simulink model "sysgenCORDICSinCos"  (Simulink 7.7)
settings: Solver=ode45  StartTime=0.0  StopTime=500  RelTol=1e-3
values from neighbouring files (symbols this model uses):
  blue = blue(1:(min_x*min_y))    [makematrix.m]    (also in rgb.mat = [0 0 0 255 255 255 255 255 255 0 0 0 ... (256 elements, 256x)
undefined symbols (not defined in the file or in its folder): Error_Measurement, sysgenCORDIC_lib
libraries: xbsIndex_r4 x95, dspobslib x9, dspstat3 x4, dspswit3 x2, xbsCopyrightNotice_r4 x1, simulink x1
(part 2 of 2)

== system sysgenCORDICSinCos/SINCOS testbench/SinCos/fine_angle_pe/cordic_pe7 ==
  xi : Inport
  yi : Inport  Port=2
  zi : Inport  Port=3
  AddSub22 : xbsIndex_r4/AddSub  mode=Addition or Subtraction  use_carryin=off  use_carryout=off  en=off  latency=1  precision=User Defined  arith_type="Signed  (2's comp)"  n_bits=16  bin_pt=13  quantization=Truncate  overflow=Wrap  dbl_ovrd=off  use_behavioral_HDL=off  hw_selection=Fabric  pipelined=off  block_type=addsub
  AddSub23 : xbsIndex_r4/AddSub  mode=Addition or Subtraction  use_carryin=off  use_carryout=off  en=off  latency=1  precision=User Defined  arith_type="Signed  (2's comp)"  n_bits=16  bin_pt=13  quantization=Truncate  overflow=Wrap  dbl_ovrd=off  use_behavioral_HDL=off  hw_selection=Fabric  pipelined=off  block_type=addsub
  AddSub24 : xbsIndex_r4/AddSub  mode=Addition or Subtraction  use_carryin=off  use_carryout=off  en=off  latency=1  precision=User Defined  arith_type="Signed  (2's comp)"  n_bits=16  bin_pt=13  quantization=Truncate  overflow=Wrap  dbl_ovrd=off  use_behavioral_HDL=off  hw_selection=Fabric  pipelined=off  block_type=addsub
  Constant11 : xbsIndex_r4/Constant  const=0.00781234106010111  gui_display_data_type=Fixed-point  arith_type=Signed (2's comp)  n_bits=16  bin_pt=13  preci_type=Single  exp_width=8  frac_width=24  explicit_period=off  period=1  equ=P=C  opselect=C  inp2=PCIN>>17  opr=+  inp1=P  carry=CIN  dbl_ovrd=off  block_type=constant
  Inverter8 : xbsIndex_r4/Inverter  en=off  latency=0  dbl_ovrd=off  block_type=inv
  Shift14 : xbsIndex_r4/Shift  shift_dir=Right  shift_bits=7  en=off  latency=0  precision=User Defined  arith_type="Signed  (2's comp)"  n_bits=16  bin_pt=13  quantization=Truncate  overflow=Wrap  dbl_ovrd=off  block_type=shift
  Shift15 : xbsIndex_r4/Shift  shift_dir=Right  shift_bits=7  en=off  latency=0  precision=User Defined  arith_type="Signed  (2's comp)"  n_bits=16  bin_pt=13  quantization=Truncate  overflow=Wrap  dbl_ovrd=off  block_type=shift
  Slice9 : xbsIndex_r4/Slice  nbits=1  boolean_output=on  mode=Upper Bit Location + Width  bit1=0  base1=MSB of Input  bit0=0  base0=LSB of Input  dbl_ovrd=off  block_type=slice
  xo : Outport
  yo : Outport  Port=2
  zo : Outport  Port=3
  wires:
  xi/1 -> AddSub22/1, Shift14/1
  yi/1 -> AddSub23/1, Shift15/1
  zi/1 -> AddSub24/1, Slice9/1
  Slice9/1 -> AddSub23/3, Inverter8/1
  Inverter8/1 -> AddSub24/3, AddSub22/3
  AddSub24/1 -> zo/1
  Constant11/1 -> AddSub24/2
  AddSub23/1 -> yo/1
  Shift14/1 -> AddSub23/2
  AddSub22/1 -> xo/1
  Shift15/1 -> AddSub22/2
